simulink model "control"  (R2021a)
settings: Solver=VariableStepAuto  StartTime=0.0  StopTime=10.0  RelTol=1e-3
settings Model: Creator=11062  LastModifiedBy=11062

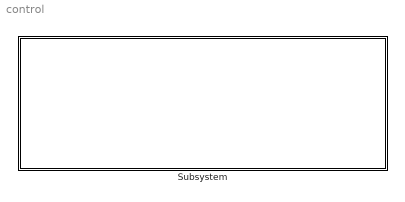
== system control ==
  Subsystem : Subsystem

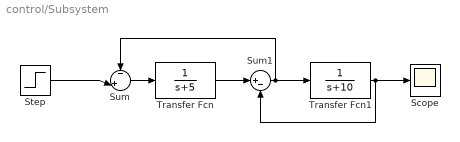
== system control/Subsystem ==
  Scope : Scope
  Step : Step  SampleTime=0
  Sum : Sum  Inputs=-|+|
  Sum1 : Sum  Inputs=|+-
  Transfer Fcn : TransferFcn  Denominator=[1 5]
  Transfer Fcn1 : TransferFcn  Denominator=[1 10]
  wires:
  Transfer Fcn1/1 -> Sum1/2, Scope/1
  Transfer Fcn/1 -> Sum1/1
  Sum1/1 -> Sum/1, Transfer Fcn1/1
  Sum/1 -> Transfer Fcn/1
  Step/1 -> Sum/2
